simulink model "TEST_LIDAR"  (R2022b)
settings: Solver=FixedStepAuto  StartTime=0.0  StopTime=inf  FixedStep=1e-3  RelTol=1e-3  EnableMultiTasking=on
model workspace (MAT data in the model file):
  SL_ROS_VariableLengthArrays_MaxSizes : object (value not decoded)
values from neighbouring files (symbols this model uses):
  data = theClient.GetLastFrameOfData()    [FuncMotive.m]
undefined symbols (not defined in the file or in its folder): angular, carstamp, CIRCUIT, CLTF_DAMP, CLTF_FREQ, CLTF_GAIN, CONTROL, CONTROL_INI, DiscIntNeverNeededParam, INPUT, linear, MCP3201, MD25, MODEL, MODEL_INI, mpcstate, MPU60X0, MPU9250, MSG, NAV_MPC_CONTROL, OUTPUT, RCRX, SAMPLING_TIME, SYSID_INPUT, VL6180X
libraries: raspberrypiCommlib x160, simulink x89, raspberrypiNetworklib x22, ros2lib x14, dspsigattribs x14, embedlinuxBasiclib x12, ctrlSharedLib x2, mpclib x1, vrlib x1, sldrtlib x1
(part 4 of 19)

== system TEST_LIDAR/GAZEBO SIMULATION/COMMUNICATIONS/TCP//IP NAV ==
  Bus Selector : BusSelector  OutputSignals=INPUT.NAV_EARTH_POS,INPUT.NAV_EULER_ANG
  Data Store Read2 : DataStoreRead  DataStoreName=CONTROL  SampleTime=SAMPLING_TIME  IndexOptions=Index vector (dialog)  Indices=1  OutputSizes=1
  Data Store Write1 : DataStoreWrite  DataStoreName=CONTROL  DataStoreElements=CONTROL.STATE.NAV_RX_STATUS  IndexOptions=Index vector (dialog)  Indices=1  OutputSizes=1
  Data Store Write2 : DataStoreWrite  DataStoreName=CONTROL  IndexOptions=Index vector (dialog)  Indices=1  OutputSizes=1
  Data Type Conversion : DataTypeConversion  OutDataTypeStr=uint8  SaturateOnIntegerOverflow=off  RndMeth=Floor
  Display{,1..3} (4 alike) : Display
  NAV RX : MATLAB Function  Priority=20  TreatAsAtomicUnit=on
  NAV_EARTH_POS : Scope
  NAV_EULER_ANG : Scope
  TCP/IP Receive : raspberrypiNetworklib/TCP//IP Receive  Mode_=Server  LocalServerPort_=3000  RemoteAddr_=127.0.0.1  RemoteServerPort_=3000  DataType_=uint8  DataSize_=24  SampleTime_=SAMPLING_TIME  SimulateUsing=Code generation  ClientPortBindingSelection_=off  ClientPortToBind_=35000  BlockingMode_=off  BlockTimeout_=0.1  BlockPlatform=RASPBERRYPI
  wires:
  NAV RX/1(CONTROL) -> Bus Selector/1, Data Store Write2/1
  Data Store Read2/1 -> NAV RX/1(CONTROL_IN)
  TCP/IP Receive/1 -> NAV RX/2(PAYLOAD), Display1/1
  Bus Selector/1 -> NAV_EARTH_POS/1, Display2/1  "<NAV_EARTH_POS>"
  Bus Selector/2 -> NAV_EULER_ANG/1, Display3/1  "<NAV_EULER_ANG>"
  Data Type Conversion/1 -> Data Store Write1/1, Display/1, NAV RX/3(STATUS)
  TCP/IP Receive/2 -> Data Type Conversion/1

== system TEST_LIDAR/GAZEBO SIMULATION/COMMUNICATIONS/TCP//IP SLAM ==
  Data Store Read1 : DataStoreRead  DataStoreName=CONTROL  SampleTime=SAMPLING_TIME  IndexOptions=Index vector (dialog)  Indices=1  OutputSizes=1
  SLAM TX : MATLAB Function  Priority=20  TreatAsAtomicUnit=on
  TCP/IP Send : raspberrypiNetworklib/TCP//IP Send  Mode_=Server  LocalServerPort_=7001  RemoteAddr_=127.0.0.1  RemoteServerPort_=25000  SimulateUsing=Code generation  ClientPortBindingSelection_=off  ClientPortToBind_=35000  BlockingMode_=off  BlockTimeout_=0.1  BlockPlatform=RASPBERRYPI
  wires:
  SLAM TX/1(PAYLOAD) -> TCP/IP Send/1
  Data Store Read1/1 -> SLAM TX/1(CONTROL)

== system TEST_LIDAR/GAZEBO SIMULATION/COMMUNICATIONS/TCP//IP TEST ==
  Constant : Constant  Value=127  OutDataTypeStr=uint8  SampleTime=SAMPLING_TIME
  Data Type Conversion : DataTypeConversion  OutDataTypeStr=uint8  SaturateOnIntegerOverflow=off  RndMeth=Floor
  Display2 : Display
  Display3 : Display
  TCP/IP Receive : raspberrypiNetworklib/TCP//IP Receive  Mode_=Client  LocalServerPort_=3000  RemoteAddr_=192.168.1.21  RemoteServerPort_=27000  DataType_=uint8  DataSize_=1  SampleTime_=SAMPLING_TIME  SimulateUsing=Code generation  ClientPortBindingSelection_=off  ClientPortToBind_=35000  BlockingMode_=off  BlockTimeout_=0.1  BlockPlatform=RASPBERRYPI
  TCP/IP Send : raspberrypiNetworklib/TCP//IP Send  Mode_=Server  LocalServerPort_=27000  RemoteAddr_=127.0.0.1  RemoteServerPort_=25000  SimulateUsing=Code generation  ClientPortBindingSelection_=off  ClientPortToBind_=35000  BlockingMode_=off  BlockTimeout_=0.1  BlockPlatform=RASPBERRYPI
  wires:
  TCP/IP Receive/2 -> Data Type Conversion/1
  Data Type Conversion/1 -> Display3/1
  Constant/1 -> TCP/IP Send/1
  TCP/IP Receive/1 -> Display2/1

== system TEST_LIDAR/GAZEBO SIMULATION/COMMUNICATIONS/UART ==
  Compare To Zero : simulink/Logic and Bit Operations/Compare To Zero  relop=>  OutDataTypeStr=boolean
  Data Store Read : DataStoreRead  DataStoreName=CONTROL  SampleTime=SAMPLING_TIME  DataStoreElements=CONTROL.STATE.UART_MODE  IndexOptions=Index vector (dialog)  Indices=1  OutputSizes=1
  MSG_RX : Subsystem  Priority=10
      settings: RTWSystemCode=Nonreusable function  FunctionWithSeparateData=on
  MSG_TX : Subsystem  Priority=10
      settings: RTWSystemCode=Nonreusable function  FunctionWithSeparateData=on
  wires:
  Data Store Read/1 -> Compare To Zero/1
  Compare To Zero/1 -> MSG_TX/Enable

== system TEST_LIDAR/GAZEBO SIMULATION/COMMUNICATIONS/UART_MUX ==
  A : embedlinuxBasiclib/GPIO Write  Priority=4  board=Pi 3 Model B+  gpio=8  direction=Output  blockPlatform=Raspberry Pi
  B : embedlinuxBasiclib/GPIO Write  Priority=5  board=Pi 3 Model B+  gpio=18  direction=Output  blockPlatform=Raspberry Pi
  BT MCS : Subsystem  Priority=1
      settings: RTWSystemCode=Nonreusable function  FunctionWithSeparateData=on
  INH : embedlinuxBasiclib/GPIO Write  Priority=6  board=Pi 3 Model B+  gpio=5  direction=Output  blockPlatform=Raspberry Pi
  MATLAB Function : MATLAB Function  Priority=3  TreatAsAtomicUnit=on
  RCRX iBUS : Subsystem  Priority=2
  Serial Read : raspberrypiCommlib/Serial Read  Priority=0  board=Pi 3 Model B+  SCIModule_=/dev/ttyS0  Baudrate_=57600  Parity=None  StopBits_=1  HardwareFlowControl=None  ByteOrder=LittleEndian  DataLength=50  DataType=uint8  OutputStatus=on  SampleTime=SAMPLING_TIME  blockPlatform=RaspberryPi
  Terminator : Terminator
  wires:
  Serial Read/1 -> BT MCS/1(Data), RCRX iBUS/1(Data)
  Serial Read/2 -> Terminator/1
  MATLAB Function/5(BL) -> BT MCS/Enable
  MATLAB Function/4(RCRX) -> RCRX iBUS/Enable
  MATLAB Function/3(INH) -> INH/1
  MATLAB Function/2(B) -> B/1
  MATLAB Function/1(A) -> A/1

== system TEST_LIDAR/GAZEBO SIMULATION/COMMUNICATIONS/UDP//ROS ==
  Compare To Zero : simulink/Logic and Bit Operations/Compare To Zero  relop=>  OutDataTypeStr=boolean
  Data Store Read : DataStoreRead  DataStoreName=MSG  SampleTime=SAMPLING_TIME  DataStoreElements=MSG.TX_BUFFER(1,1)  IndexOptions=Index vector (dialog)  Indices=1  OutputSizes=1
  MSG_RX : Subsystem  Priority=10  TreatAsAtomicUnit=on
      settings: RTWSystemCode=Nonreusable function  FunctionWithSeparateData=on
  MSG_TX : Subsystem  Priority=10
      settings: RTWSystemCode=Nonreusable function  FunctionWithSeparateData=on
  wires:
  Compare To Zero/1 -> MSG_TX/Enable
  Data Store Read/1 -> Compare To Zero/1

== system TEST_LIDAR/GAZEBO SIMULATION/SENSORS/READ IMU ==
  " LPF 3" : Subsystem
  " LPF 4" : Subsystem
  Bus Selector : BusSelector  OutputSignals=linear_acceleration.x,linear_acceleration.y,linear_acceleration.z,angular_velocity.x,angular_velocity.y,angular_velocity.z
  Constant2 : Constant  Value=MPU60X0.ACCEL_CALIB  SampleTime=MPU60X0.SAMPLING_TIME
  Constant3 : Constant  Value=CONTROL_INI.PARAM.GRAVITY  SampleTime=MPU60X0.SAMPLING_TIME
  Constant4 : Constant  Value=MPU60X0.ALFA_CALIB  SampleTime=MPU60X0.SAMPLING_TIME
  Data Store Memory1 : DataStoreMemory  Priority=10  DataStoreName=MPU60X0_PITCH_OFFS  ReadBeforeWriteMsg=warning  WriteAfterWriteMsg=warning  WriteAfterReadMsg=warning  ShowAdditionalParam=off  OutDataTypeStr=double
  Data Store Memory5 : DataStoreMemory  Priority=10  DataStoreName=MPU60X0_ACCEL_OFFS  ReadBeforeWriteMsg=warning  WriteAfterWriteMsg=warning  WriteAfterReadMsg=warning  InitialValue=zeros(3,1)  ShowAdditionalParam=off  OutDataTypeStr=double
  Data Store Memory6 : DataStoreMemory  Priority=10  DataStoreName=MPU60X0_GYRO_OFFS  ReadBeforeWriteMsg=warning  WriteAfterWriteMsg=warning  WriteAfterReadMsg=warning  InitialValue=zeros(3,1)  ShowAdditionalParam=off  OutDataTypeStr=double
  Data Store Read : DataStoreRead  DataStoreName=CONTROL  SampleTime=MPU60X0.SAMPLING_TIME  DataStoreElements=CONTROL.STATE.VEHICLE_MODE  IndexOptions=Index vector (dialog)  Indices=1  OutputSizes=1
  Data Store Read1 : DataStoreRead  DataStoreName=MPU60X0_PITCH_OFFS  SampleTime=MPU60X0.SAMPLING_TIME  IndexOptions=Index vector (dialog)  Indices=1  OutputSizes=1
  Data Store Read6 : DataStoreRead  DataStoreName=MPU60X0_ACCEL_OFFS  SampleTime=MPU60X0.SAMPLING_TIME  IndexOptions=Index vector (dialog)  Indices=1  OutputSizes=1
  Data Store Read8 : DataStoreRead  DataStoreName=MPU60X0_GYRO_OFFS  SampleTime=MPU60X0.SAMPLING_TIME  IndexOptions=Index vector (dialog)  Indices=1  OutputSizes=1
  Data Store Read9 : DataStoreRead  DataStoreName=CONTROL  SampleTime=MPU60X0.SAMPLING_TIME  IndexOptions=Index vector (dialog)  Indices=1  OutputSizes=1
  Data Store Write3 : DataStoreWrite  DataStoreName=MPU60X0_ACCEL_OFFS  IndexOptions=Index vector (dialog)  Indices=1  OutputSizes=1
  Data Store Write4 : DataStoreWrite  DataStoreName=MPU60X0_GYRO_OFFS  IndexOptions=Index vector (dialog)  Indices=1  OutputSizes=1
  Data Store Write5 : DataStoreWrite  DataStoreName=CONTROL  IndexOptions=Index vector (dialog)  Indices=1  OutputSizes=1
  FILTER POLE : Subsystem
  GRAVITY ROTATION : MATLAB Function  TreatAsAtomicUnit=on
  IMU CALIBRATION : MATLAB Function  Priority=30  TreatAsAtomicUnit=on
  LPF 1 : Subsystem
  "LPF 2 " : Subsystem
  MEAN FILTER : DiscreteFilter  Numerator=1/floor(SAMPLING_TIME*1000)*ones(1,floor(SAMPLING_TIME*1000))  Denominator=[1 zeros(1,floor(SAMPLING_TIME*1000)-1)]
  "MEAN FILTER " : DiscreteFilter  Numerator=1/floor(SAMPLING_TIME*1000)*ones(1,floor(SAMPLING_TIME*1000))  Denominator=[1 zeros(1,floor(SAMPLING_TIME*1000)-1)]
  Mux : Mux  Inputs=3
  Mux1 : Mux  Inputs=3
  Scope : Scope  NumInputPorts=2
  Subscribe : ros2lib/Subscribe  topicSource=Specify your own  topic=/imu  messageType=sensor_msgs/Imu  sampleTime=-1  QOSHistory=Keep last  QOSDepth=1  QOSReliability=Reliable  QOSDurability=Volatile
      settings: LibrarySourceBlock=roslib/ROS 2/Subscribe
  Terminator : Terminator
  wires:
  Constant4/1 -> IMU CALIBRATION/11(ALFA_CALIB)
  Constant2/1 -> IMU CALIBRATION/10(ACCEL_CALIB)
  FILTER POLE/1(ALFA) -> " LPF 4"/2(ALFA), " LPF 3"/2(ALFA), LPF 1/2(ALFA), "LPF 2 "/2(ALFA)
  Mux1/1 -> "MEAN FILTER "/1, IMU CALIBRATION/6(GYRO), " LPF 3"/1(IN), Scope/2
  LPF 1/1(OUT) -> IMU CALIBRATION/3(ACCEL_FILT)
  " LPF 3"/1(OUT) -> IMU CALIBRATION/7(GYRO_FILT)
  " LPF 4"/1(OUT) -> IMU CALIBRATION/9(GYRO_MEAN_FILT)
  Data Store Read9/1 -> IMU CALIBRATION/1(CONTROL_IN)
  "LPF 2 "/1(OUT) -> IMU CALIBRATION/5(ACCEL_MEAN_FILT)
  IMU CALIBRATION/3(GYRO_OFFS_OUT) -> Data Store Write4/1
  Data Store Read6/1 -> IMU CALIBRATION/12(ACCEL_OFFS_IN)
  IMU CALIBRATION/1(CONTROL) -> Data Store Write5/1
  MEAN FILTER/1 -> "LPF 2 "/1(IN), IMU CALIBRATION/4(ACCEL_MEAN)
  Data Store Read8/1 -> IMU CALIBRATION/13(GYRO_OFFS_IN)
  IMU CALIBRATION/2(ACCEL_OFFS_OUT) -> Data Store Write3/1
  "MEAN FILTER "/1 -> IMU CALIBRATION/8(GYRO_MEAN), " LPF 4"/1(IN)
  Mux/1 -> Scope/1, IMU CALIBRATION/2(ACCEL), LPF 1/1(IN), MEAN FILTER/1
  Constant3/1 -> GRAVITY ROTATION/2(GRAVITY)
  Data Store Read1/1 -> GRAVITY ROTATION/1(PITCH_OFFSET)
  GRAVITY ROTATION/1(GRAVITY_VECTOR) -> IMU CALIBRATION/14(GRAVITY_VECTOR)
  Data Store Read/1 -> GRAVITY ROTATION/3(VEHICLE_MODE)
  Subscribe/2 -> Bus Selector/1
  Subscribe/1 -> Terminator/1
  Bus Selector/1 -> Mux/1  "<x>"
  Bus Selector/2 -> Mux/2  "<y>"
  Bus Selector/3 -> Mux/3  "<z>"
  Bus Selector/4 -> Mux1/1  "<x>"
  Bus Selector/5 -> Mux1/2  "<y>"
  Bus Selector/6 -> Mux1/3  "<z>"

== system TEST_LIDAR/GAZEBO SIMULATION/SENSORS/READ MOTOR ENCODER ==
  Bus Selector : BusSelector  OutputSignals=data
  Bus Selector1 : BusSelector  OutputSignals=data
  Bus Selector2 : BusSelector  OutputSignals=INPUT.FORWARD_VEL,INPUT.YAW_RATE
  Data Store Read : DataStoreRead  DataStoreName=CONTROL  SampleTime=SAMPLING_TIME  IndexOptions=Index vector (dialog)  Indices=1  OutputSizes=1
  Data Store Write1 : DataStoreWrite  DataStoreName=CONTROL  IndexOptions=Index vector (dialog)  Indices=1  OutputSizes=1
  MATLAB Function : MATLAB Function  TreatAsAtomicUnit=on
  Mux : Mux  Inputs=2
  Mux1 : Mux  Inputs=2
  READ_ENCODER : MATLAB Function  TreatAsAtomicUnit=on
  Scope : Scope  NumInputPorts=3
  Subscribe : ros2lib/Subscribe  topicSource=Select from ROS network  topic=/model/FullKitt/right_wheel_joint/motor_encoder  messageType=std_msgs/Int32  sampleTime=-1  QOSHistory=Keep last  QOSDepth=1  QOSReliability=Reliable  QOSDurability=Volatile
      settings: LibrarySourceBlock=roslib/ROS 2/Subscribe
  Subscribe1 : ros2lib/Subscribe  topicSource=Select from ROS network  topic=/model/FullKitt/left_wheel_joint/motor_encoder  messageType=std_msgs/Int32  sampleTime=-1  QOSHistory=Keep last  QOSDepth=1  QOSReliability=Reliable  QOSDurability=Volatile
      settings: LibrarySourceBlock=roslib/ROS 2/Subscribe
  wires:
  Data Store Read/1 -> READ_ENCODER/1(CONTROL_IN)
  READ_ENCODER/1(CONTROL) -> Bus Selector2/1, Data Store Write1/1
  Subscribe/2 -> Bus Selector/1
  Subscribe1/2 -> Bus Selector1/1
  Bus Selector/1 -> MATLAB Function/1(right_enc), Mux/1, READ_ENCODER/2(right_enc)  "<data>"
  Bus Selector1/1 -> MATLAB Function/2(left_enc), Mux/2, READ_ENCODER/3(left_enc)  "<data>"
  Bus Selector2/1 -> Mux1/2  "<FORWARD_VEL>"
  Bus Selector2/2 -> Scope/2  "<YAW_RATE>"
  Mux/1 -> Scope/3
  Mux1/1 -> Scope/1
  MATLAB Function/1(avg_encoder) -> Mux1/1

== system TEST_LIDAR/GAZEBO SIMULATION/SENSORS/WALL RANGE SENSOR ==
  ANGLE AND DISTANCE COMPUTATION : Subsystem  TreatAsAtomicUnit=on
      settings: MinAlgLoopOccurrences=on
  Data Store Memory : DataStoreMemory  DataStoreName=REAR_DISTANCE  ReadBeforeWriteMsg=warning  WriteAfterWriteMsg=warning  WriteAfterReadMsg=warning  ShowAdditionalParam=off  OutDataTypeStr=double
  Data Store Memory1 : DataStoreMemory  DataStoreName=FRONT_DISTANCE  ReadBeforeWriteMsg=warning  WriteAfterWriteMsg=warning  WriteAfterReadMsg=warning  ShowAdditionalParam=off  OutDataTypeStr=double
  FRONT : Subsystem  TreatAsAtomicUnit=on
      settings: MinAlgLoopOccurrences=on  RTWSystemCode=Nonreusable function  FunctionWithSeparateData=on
  REAR : Subsystem  TreatAsAtomicUnit=on
      settings: MinAlgLoopOccurrences=on  RTWSystemCode=Nonreusable function  FunctionWithSeparateData=on

== system TEST_LIDAR/HARDWARE/ACTUATORS/MD25_I2C ==
  Cast : DataTypeConversion  OutDataTypeStr=uint8  SaturateOnIntegerOverflow=off  RndMeth=Floor
  Compare To Constant : simulink/Logic and Bit Operations/Compare To Constant  relop===  const=0  OutDataTypeStr=uint8
  Data Store Memory : DataStoreMemory  Priority=10  DataStoreName=MD25_INIT  ReadBeforeWriteMsg=warning  WriteAfterWriteMsg=warning  WriteAfterReadMsg=warning  ShowAdditionalParam=off  OutDataTypeStr=boolean
  Data Store Read : DataStoreRead  DataStoreName=MD25_INIT  SampleTime=SAMPLING_TIME  IndexOptions=Index vector (dialog)  Indices=1  OutputSizes=1
  Data Store Read1 : DataStoreRead  DataStoreName=MD25_INIT  IndexOptions=Index vector (dialog)  Indices=1  OutputSizes=1
  Data Store Read2 : DataStoreRead  DataStoreName=CONTROL  SampleTime=SAMPLING_TIME  DataStoreElements=CONTROL.STATE.CURRENT_STATUS_SYS  IndexOptions=Index vector (dialog)  Indices=1  OutputSizes=1
  Data Store Write : DataStoreWrite  DataStoreName=CONTROL  DataStoreElements=CONTROL.STATE.MD25_INIT  IndexOptions=Index vector (dialog)  Indices=1  OutputSizes=1
  Logical Operator : Logic  Operator=NOT  AllPortsSameDT=off  OutDataTypeStr=boolean
  MD25 INITIALIZATION : Subsystem  Priority=10
      settings: RTWSystemCode=Nonreusable function
  READ BATTERY VOLTAGE : Subsystem  Priority=20  TreatAsAtomicUnit=on
      settings: RTWSystemCode=Nonreusable function
  READ MOTOR CURRENT : Subsystem  Priority=30  TreatAsAtomicUnit=on
      settings: RTWSystemCode=Nonreusable function
  READ MOTOR ENCODER : Subsystem  Priority=40  TreatAsAtomicUnit=on
      settings: RTWSystemCode=Nonreusable function
  RESET MOTOR ENCODER : Subsystem  Priority=50  TreatAsAtomicUnit=on
      settings: RTWSystemCode=Nonreusable function
  "WRITE PWM MOTOR " : Subsystem  Priority=50  TreatAsAtomicUnit=on
      settings: RTWSystemCode=Nonreusable function
  wires:
  Logical Operator/1 -> MD25 INITIALIZATION/Enable
  Data Store Read1/1 -> Cast/1
  Cast/1 -> Data Store Write/1
  Data Store Read/1 -> "WRITE PWM MOTOR "/Enable, READ MOTOR ENCODER/Enable, READ MOTOR CURRENT/Enable, READ BATTERY VOLTAGE/Enable, Logical Operator/1
  Data Store Read2/1 -> Compare To Constant/1
  Compare To Constant/1 -> RESET MOTOR ENCODER/Enable

== system TEST_LIDAR/HARDWARE/ACTUATORS/RGB ==
  BLUE : embedlinuxBasiclib/GPIO Write  board=Pi 3 Model B+  gpio=25  direction=Output  blockPlatform=Raspberry Pi
  Cast1 : DataTypeConversion  OutDataTypeStr=boolean  SaturateOnIntegerOverflow=off  RndMeth=Floor
  Cast2 : DataTypeConversion  OutDataTypeStr=boolean  SaturateOnIntegerOverflow=off  RndMeth=Floor
  Cast3 : DataTypeConversion  OutDataTypeStr=boolean  SaturateOnIntegerOverflow=off  RndMeth=Floor
  Data Store Read : DataStoreRead  DataStoreName=CONTROL  SampleTime=SAMPLING_TIME  DataStoreElements=CONTROL.OUTPUT.LEDS(:,:)  IndexOptions=Index vector (dialog)  Indices=1  OutputSizes=1
  Demux : Demux  Outputs=3
  GREEN : embedlinuxBasiclib/GPIO Write  board=Pi 3 Model B+  gpio=24  direction=Output  blockPlatform=Raspberry Pi
  RED : embedlinuxBasiclib/GPIO Write  board=Pi 3 Model B+  gpio=23  direction=Output  blockPlatform=Raspberry Pi
  wires:
  Data Store Read/1 -> Demux/1
  Demux/1 -> Cast1/1
  Demux/2 -> Cast2/1
  Demux/3 -> Cast3/1
  Cast1/1 -> RED/1
  Cast2/1 -> GREEN/1
  Cast3/1 -> BLUE/1

== system TEST_LIDAR/HARDWARE/COMMUNICATIONS/BT_RX ==
  Bus Selector : BusSelector  OutputSignals=INPUT.MCS_EARTH_POS,INPUT.MCS_EULER_ANG
  Data Store Read2 : DataStoreRead  DataStoreName=CONTROL  SampleTime=SAMPLING_TIME  IndexOptions=Index vector (dialog)  Indices=1  OutputSizes=1
  Data Store Write1 : DataStoreWrite  DataStoreName=CONTROL  DataStoreElements=CONTROL.STATE.MCS_RX_STATUS  IndexOptions=Index vector (dialog)  Indices=1  OutputSizes=1
  Data Store Write2 : DataStoreWrite  DataStoreName=CONTROL  IndexOptions=Index vector (dialog)  Indices=1  OutputSizes=1
  Data Type Conversion : DataTypeConversion  OutDataTypeStr=uint8  SaturateOnIntegerOverflow=off  RndMeth=Floor
  Display{,1..3} (4 alike) : Display
  MCS RX : MATLAB Function  Priority=20  TreatAsAtomicUnit=on
  MCS_EARTH_POS : Scope
  MCS_EULER_ANG : Scope
  Serial Read : raspberrypiCommlib/Serial Read  board=Pi 3 Model B+  SCIModule_=/dev/ttyUSB0  Baudrate_=115200  Parity=None  StopBits_=1  HardwareFlowControl=None  ByteOrder=LittleEndian  DataLength=50  DataType=uint8  OutputStatus=on  SampleTime=SAMPLING_TIME  blockPlatform=RaspberryPi
  wires:
  MCS RX/1(CONTROL) -> Bus Selector/1, Data Store Write2/1
  Data Store Read2/1 -> MCS RX/1(CONTROL_IN)
  Serial Read/1 -> Display1/1, MCS RX/2(BUFFER_RX_LAST)
  Serial Read/2 -> Data Type Conversion/1
  Bus Selector/1 -> MCS_EARTH_POS/1, Display2/1  "<MCS_EARTH_POS>"
  Bus Selector/2 -> MCS_EULER_ANG/1, Display3/1  "<MCS_EULER_ANG>"
  Data Type Conversion/1 -> Data Store Write1/1, Display/1, MCS RX/3(STATUS)

== system TEST_LIDAR/HARDWARE/COMMUNICATIONS/TCP//IP ==
  Compare To Zero : simulink/Logic and Bit Operations/Compare To Zero  relop=>  OutDataTypeStr=boolean
  Data Store Read : DataStoreRead  DataStoreName=MSG  SampleTime=SAMPLING_TIME  DataStoreElements=MSG.TX_BUFFER(1,1)  IndexOptions=Index vector (dialog)  Indices=1  OutputSizes=1
  MSG_RX : Subsystem  Priority=10  TreatAsAtomicUnit=on
      settings: RTWSystemCode=Nonreusable function  FunctionWithSeparateData=on
  MSG_TX : Subsystem  Priority=10
      settings: RTWSystemCode=Nonreusable function  FunctionWithSeparateData=on
  wires:
  Compare To Zero/1 -> MSG_TX/Enable
  Data Store Read/1 -> Compare To Zero/1

== system TEST_LIDAR/HARDWARE/COMMUNICATIONS/TCP//IP LIDAR ==
  Bus Selector : BusSelector  OutputSignals=INPUT.LIDAR_2D
  Data Store Read1 : DataStoreRead  DataStoreName=CONTROL  SampleTime=SAMPLING_TIME  DataStoreElements=CONTROL.STATE.LIDAR_2D_MODE  IndexOptions=Index vector (dialog)  Indices=1  OutputSizes=1
  Data Store Read2 : DataStoreRead  DataStoreName=CONTROL  SampleTime=SAMPLING_TIME  IndexOptions=Index vector (dialog)  Indices=1  OutputSizes=1
  Data Store Write1 : DataStoreWrite  DataStoreName=CONTROL  DataStoreElements=CONTROL.STATE.NAV_RX_STATUS  IndexOptions=Index vector (dialog)  Indices=1  OutputSizes=1
  Data Store Write2 : DataStoreWrite  DataStoreName=CONTROL  IndexOptions=Index vector (dialog)  Indices=1  OutputSizes=1
  Data Type Conversion : DataTypeConversion  OutDataTypeStr=uint8  SaturateOnIntegerOverflow=off  RndMeth=Floor
  Display : Display
  Display1 : Display
  Display2 : Display
  NAV RX : MATLAB Function  Priority=20  TreatAsAtomicUnit=on
  TCP/IP Receive : raspberrypiNetworklib/TCP//IP Receive  Mode_=Server  LocalServerPort_=7000  RemoteAddr_=127.0.0.1  RemoteServerPort_=3000  DataType_=uint8  DataSize_=160  SampleTime_=SAMPLING_TIME  SimulateUsing=Code generation  ClientPortBindingSelection_=off  ClientPortToBind_=35000  BlockingMode_=off  BlockTimeout_=0.1  BlockPlatform=RASPBERRYPI
  TCP/IP Send : raspberrypiNetworklib/TCP//IP Send  Mode_=Server  LocalServerPort_=7001  RemoteAddr_=127.0.0.1  RemoteServerPort_=25000  SimulateUsing=Code generation  ClientPortBindingSelection_=off  ClientPortToBind_=35000  BlockingMode_=off  BlockTimeout_=0.1  BlockPlatform=RASPBERRYPI
  wires:
  NAV RX/1(CONTROL) -> Bus Selector/1, Data Store Write2/1
  Data Store Read2/1 -> NAV RX/1(CONTROL_IN)
  TCP/IP Receive/1 -> NAV RX/2(PAYLOAD), Display1/1
  Bus Selector/1 -> Display2/1  "<LIDAR_2D>"
  Data Type Conversion/1 -> Data Store Write1/1, Display/1, NAV RX/3(STATUS)
  TCP/IP Receive/2 -> Data Type Conversion/1
  Data Store Read1/1 -> TCP/IP Send/1

== system TEST_LIDAR/HARDWARE/COMMUNICATIONS/TCP//IP MCS ==
  Bus Selector : BusSelector  OutputSignals=INPUT.MCS_EARTH_POS,INPUT.MCS_EULER_ANG
  Data Store Read2 : DataStoreRead  DataStoreName=CONTROL  SampleTime=SAMPLING_TIME  IndexOptions=Index vector (dialog)  Indices=1  OutputSizes=1
  Data Store Write1 : DataStoreWrite  DataStoreName=CONTROL  DataStoreElements=CONTROL.STATE.MCS_RX_STATUS  IndexOptions=Index vector (dialog)  Indices=1  OutputSizes=1
  Data Store Write2 : DataStoreWrite  DataStoreName=CONTROL  IndexOptions=Index vector (dialog)  Indices=1  OutputSizes=1
  Data Type Conversion : DataTypeConversion  OutDataTypeStr=uint8  SaturateOnIntegerOverflow=off  RndMeth=Floor
  Display{,1..3} (4 alike) : Display
  MCS RX : MATLAB Function  Priority=20  TreatAsAtomicUnit=on
  MCS_EARTH_POS : Scope
  MCS_EULER_ANG : Scope
  TCP/IP Receive : raspberrypiNetworklib/TCP//IP Receive  Mode_=Server  LocalServerPort_=15000  RemoteAddr_=127.0.0.1  RemoteServerPort_=3000  DataType_=uint8  DataSize_=26  SampleTime_=SAMPLING_TIME  SimulateUsing=Code generation  ClientPortBindingSelection_=off  ClientPortToBind_=35000  BlockingMode_=off  BlockTimeout_=0.1  BlockPlatform=RASPBERRYPI
  wires:
  TCP/IP Receive/2 -> Data Type Conversion/1
  Data Type Conversion/1 -> MCS RX/3(STATUS), Display/1, Data Store Write1/1
  Bus Selector/2 -> Display3/1, MCS_EULER_ANG/1  "<MCS_EULER_ANG>"
  Bus Selector/1 -> Display2/1, MCS_EARTH_POS/1  "<MCS_EARTH_POS>"
  TCP/IP Receive/1 -> Display1/1, MCS RX/2(PAYLOAD)
  Data Store Read2/1 -> MCS RX/1(CONTROL_IN)
  MCS RX/1(CONTROL) -> Data Store Write2/1, Bus Selector/1

== system TEST_LIDAR/HARDWARE/COMMUNICATIONS/TCP//IP NAV ==
  Bus Selector : BusSelector  OutputSignals=INPUT.NAV_EARTH_POS,INPUT.NAV_EULER_ANG
  Data Store Read2 : DataStoreRead  DataStoreName=CONTROL  SampleTime=SAMPLING_TIME  IndexOptions=Index vector (dialog)  Indices=1  OutputSizes=1
  Data Store Write1 : DataStoreWrite  DataStoreName=CONTROL  DataStoreElements=CONTROL.STATE.NAV_RX_STATUS  IndexOptions=Index vector (dialog)  Indices=1  OutputSizes=1
  Data Store Write2 : DataStoreWrite  DataStoreName=CONTROL  IndexOptions=Index vector (dialog)  Indices=1  OutputSizes=1
  Data Type Conversion : DataTypeConversion  OutDataTypeStr=uint8  SaturateOnIntegerOverflow=off  RndMeth=Floor
  Display{,1..3} (4 alike) : Display
  NAV RX : MATLAB Function  Priority=20  TreatAsAtomicUnit=on
  NAV_EARTH_POS : Scope
  NAV_EULER_ANG : Scope
  TCP/IP Receive : raspberrypiNetworklib/TCP//IP Receive  Mode_=Server  LocalServerPort_=3000  RemoteAddr_=127.0.0.1  RemoteServerPort_=3000  DataType_=uint8  DataSize_=24  SampleTime_=SAMPLING_TIME  SimulateUsing=Code generation  ClientPortBindingSelection_=off  ClientPortToBind_=35000  BlockingMode_=off  BlockTimeout_=0.1  BlockPlatform=RASPBERRYPI
  wires:
  NAV RX/1(CONTROL) -> Bus Selector/1, Data Store Write2/1
  Data Store Read2/1 -> NAV RX/1(CONTROL_IN)
  TCP/IP Receive/1 -> NAV RX/2(PAYLOAD), Display1/1
  Bus Selector/1 -> NAV_EARTH_POS/1, Display2/1  "<NAV_EARTH_POS>"
  Bus Selector/2 -> NAV_EULER_ANG/1, Display3/1  "<NAV_EULER_ANG>"
  Data Type Conversion/1 -> Data Store Write1/1, Display/1, NAV RX/3(STATUS)
  TCP/IP Receive/2 -> Data Type Conversion/1

== system TEST_LIDAR/HARDWARE/COMMUNICATIONS/TCP//IP RPI4 ==
  Bus Selector : BusSelector  OutputSignals=INPUT.LIDAR_2D
  Bus Selector1 : BusSelector  OutputSignals=PARAM.LIDAR_2D_MAP
  Data Store Read2 : DataStoreRead  Priority=10  DataStoreName=CONTROL  SampleTime=SAMPLING_TIME  IndexOptions=Index vector (dialog)  Indices=1  OutputSizes=1
  Data Store Read3 : DataStoreRead  Priority=40  DataStoreName=CONTROL  SampleTime=SAMPLING_TIME  IndexOptions=Index vector (dialog)  Indices=1  OutputSizes=1
  Data Store Write1 : DataStoreWrite  DataStoreName=CONTROL  DataStoreElements=CONTROL.STATE.NAV_RX_STATUS  IndexOptions=Index vector (dialog)  Indices=1  OutputSizes=1
  Data Store Write2 : DataStoreWrite  Priority=30  DataStoreName=CONTROL  IndexOptions=Index vector (dialog)  Indices=1  OutputSizes=1
  Data Type Conversion : DataTypeConversion  OutDataTypeStr=uint8  SaturateOnIntegerOverflow=off  RndMeth=Floor
  Display : Display
  Display1 : Display
  Display2 : Display
  RPI4 CODER : MATLAB Function  Priority=50  TreatAsAtomicUnit=on
  RPI4 DECODER : MATLAB Function  Priority=20  TreatAsAtomicUnit=on
  Scope : Scope
  TCP/IP Receive : raspberrypiNetworklib/TCP//IP Receive  Priority=0  Mode_=Server  LocalServerPort_=7000  RemoteAddr_=127.0.0.1  RemoteServerPort_=3000  DataType_=uint8  DataSize_=584  SampleTime_=SAMPLING_TIME  SimulateUsing=Code generation  ClientPortBindingSelection_=off  ClientPortToBind_=35000  BlockingMode_=off  BlockTimeout_=0.1  BlockPlatform=RASPBERRYPI
  TCP/IP Send : raspberrypiNetworklib/TCP//IP Send  Priority=60  Mode_=Server  LocalServerPort_=7001  RemoteAddr_=127.0.0.1  RemoteServerPort_=25000  SimulateUsing=Code generation  ClientPortBindingSelection_=off  ClientPortToBind_=35000  BlockingMode_=off  BlockTimeout_=0.1  BlockPlatform=RASPBERRYPI
  wires:
  TCP/IP Receive/2 -> Data Type Conversion/1
  Data Type Conversion/1 -> RPI4 DECODER/3(STATUS), Display/1, Data Store Write1/1
  Bus Selector/1 -> Display2/1  "<LIDAR_2D>"
  TCP/IP Receive/1 -> RPI4 DECODER/2(RX_MSG), Display1/1
  Data Store Read2/1 -> RPI4 DECODER/1(CONTROL_IN)
  RPI4 CODER/1(TX_MSG) -> TCP/IP Send/1
  Data Store Read3/1 -> RPI4 CODER/1(CONTROL)
  RPI4 DECODER/1(CONTROL) -> Bus Selector1/1, Bus Selector/1, Data Store Write2/1
  Bus Selector1/1 -> Scope/1  "<LIDAR_2D_MAP>"

== system TEST_LIDAR/HARDWARE/COMMUNICATIONS/TCP//IP SLAM ==
  Data Store Read1 : DataStoreRead  DataStoreName=CONTROL  SampleTime=SAMPLING_TIME  IndexOptions=Index vector (dialog)  Indices=1  OutputSizes=1
  SLAM TX : MATLAB Function  Priority=20  TreatAsAtomicUnit=on
  TCP/IP Send : raspberrypiNetworklib/TCP//IP Send  Mode_=Server  LocalServerPort_=7001  RemoteAddr_=127.0.0.1  RemoteServerPort_=25000  SimulateUsing=Code generation  ClientPortBindingSelection_=off  ClientPortToBind_=35000  BlockingMode_=off  BlockTimeout_=0.1  BlockPlatform=RASPBERRYPI
  wires:
  SLAM TX/1(PAYLOAD) -> TCP/IP Send/1
  Data Store Read1/1 -> SLAM TX/1(CONTROL)

== system TEST_LIDAR/HARDWARE/COMMUNICATIONS/TCP//IP TEST ==
  Constant : Constant  Value=127  OutDataTypeStr=uint8  SampleTime=SAMPLING_TIME
  Data Type Conversion : DataTypeConversion  OutDataTypeStr=uint8  SaturateOnIntegerOverflow=off  RndMeth=Floor
  Display2 : Display
  Display3 : Display
  TCP/IP Receive : raspberrypiNetworklib/TCP//IP Receive  Mode_=Client  LocalServerPort_=3000  RemoteAddr_=192.168.1.21  RemoteServerPort_=27000  DataType_=uint8  DataSize_=1  SampleTime_=SAMPLING_TIME  SimulateUsing=Code generation  ClientPortBindingSelection_=off  ClientPortToBind_=35000  BlockingMode_=off  BlockTimeout_=0.1  BlockPlatform=RASPBERRYPI
  TCP/IP Send : raspberrypiNetworklib/TCP//IP Send  Mode_=Server  LocalServerPort_=27000  RemoteAddr_=127.0.0.1  RemoteServerPort_=25000  SimulateUsing=Code generation  ClientPortBindingSelection_=off  ClientPortToBind_=35000  BlockingMode_=off  BlockTimeout_=0.1  BlockPlatform=RASPBERRYPI
  wires:
  TCP/IP Receive/2 -> Data Type Conversion/1
  Data Type Conversion/1 -> Display3/1
  Constant/1 -> TCP/IP Send/1
  TCP/IP Receive/1 -> Display2/1

== system TEST_LIDAR/HARDWARE/COMMUNICATIONS/UART ==
  Compare To Zero : simulink/Logic and Bit Operations/Compare To Zero  relop=>  OutDataTypeStr=boolean
  Data Store Read : DataStoreRead  DataStoreName=CONTROL  SampleTime=SAMPLING_TIME  DataStoreElements=CONTROL.STATE.UART_MODE  IndexOptions=Index vector (dialog)  Indices=1  OutputSizes=1
  MSG_RX : Subsystem  Priority=10
      settings: RTWSystemCode=Nonreusable function  FunctionWithSeparateData=on
  MSG_TX : Subsystem  Priority=10
      settings: RTWSystemCode=Nonreusable function  FunctionWithSeparateData=on
  wires:
  Data Store Read/1 -> Compare To Zero/1
  Compare To Zero/1 -> MSG_TX/Enable

== system TEST_LIDAR/HARDWARE/COMMUNICATIONS/UART_MUX ==
  A : embedlinuxBasiclib/GPIO Write  Priority=4  board=Pi 3 Model B+  gpio=8  direction=Output  blockPlatform=Raspberry Pi
  B : embedlinuxBasiclib/GPIO Write  Priority=5  board=Pi 3 Model B+  gpio=18  direction=Output  blockPlatform=Raspberry Pi
  BT MCS : Subsystem  Priority=1
      settings: RTWSystemCode=Nonreusable function  FunctionWithSeparateData=on
  INH : embedlinuxBasiclib/GPIO Write  Priority=6  board=Pi 3 Model B+  gpio=5  direction=Output  blockPlatform=Raspberry Pi
  MATLAB Function : MATLAB Function  Priority=3  TreatAsAtomicUnit=on
  RCRX iBUS : Subsystem  Priority=2
  Serial Read : raspberrypiCommlib/Serial Read  Priority=0  board=Pi 3 Model B+  SCIModule_=/dev/ttyS0  Baudrate_=57600  Parity=None  StopBits_=1  HardwareFlowControl=None  ByteOrder=LittleEndian  DataLength=50  DataType=uint8  OutputStatus=on  SampleTime=SAMPLING_TIME  blockPlatform=RaspberryPi
  Terminator : Terminator
  wires:
  Serial Read/1 -> BT MCS/1(Data), RCRX iBUS/1(Data)
  Serial Read/2 -> Terminator/1
  MATLAB Function/5(BL) -> BT MCS/Enable
  MATLAB Function/4(RCRX) -> RCRX iBUS/Enable
  MATLAB Function/3(INH) -> INH/1
  MATLAB Function/2(B) -> B/1
  MATLAB Function/1(A) -> A/1

== system TEST_LIDAR/HARDWARE/COMMUNICATIONS/UDP//ROS ==
  Compare To Zero : simulink/Logic and Bit Operations/Compare To Zero  relop=>  OutDataTypeStr=boolean
  Data Store Read : DataStoreRead  DataStoreName=MSG  SampleTime=SAMPLING_TIME  DataStoreElements=MSG.TX_BUFFER(1,1)  IndexOptions=Index vector (dialog)  Indices=1  OutputSizes=1
  MSG_RX : Subsystem  Priority=10  TreatAsAtomicUnit=on
      settings: RTWSystemCode=Nonreusable function  FunctionWithSeparateData=on
  MSG_TX : Subsystem  Priority=10
      settings: RTWSystemCode=Nonreusable function  FunctionWithSeparateData=on
  wires:
  Compare To Zero/1 -> MSG_TX/Enable
  Data Store Read/1 -> Compare To Zero/1

== system TEST_LIDAR/HARDWARE/SENSORS/BUTTONS ==
  BUTTON A : embedlinuxBasiclib/GPIO Read  board=Pi 3 Model B+  gpio=4  internalResistor=Off  sampleTime=SAMPLING_TIME  direction=Input  blockPlatform=Raspberry Pi
  BUTTON B : embedlinuxBasiclib/GPIO Read  board=Pi 3 Model B+  gpio=13  internalResistor=Off  sampleTime=SAMPLING_TIME  direction=Input  blockPlatform=Raspberry Pi
  BUTTON C : embedlinuxBasiclib/GPIO Read  board=Pi 3 Model B+  gpio=22  internalResistor=Off  sampleTime=SAMPLING_TIME  direction=Input  blockPlatform=Raspberry Pi
  Cast : DataTypeConversion  OutDataTypeStr=uint8  SaturateOnIntegerOverflow=off  RndMeth=Floor
  Data Store Read1 : DataStoreRead  DataStoreName=CONTROL  SampleTime=SAMPLING_TIME  DataStoreElements=CONTROL.STATE.NAV_BUTTONS(:,:)  IndexOptions=Index vector (dialog)  Indices=1  OutputSizes=1
  Data Store Read5 : DataStoreRead  DataStoreName=CONTROL  SampleTime=SAMPLING_TIME  DataStoreElements=CONTROL.STATE.PC_BUTTONS(:,:)  IndexOptions=Index vector (dialog)  Indices=1  OutputSizes=1
  Data Store Write : DataStoreWrite  DataStoreName=CONTROL  DataStoreElements=CONTROL.STATE.BUTTONS(:,:)  IndexOptions=Index vector (dialog)  Indices=1  OutputSizes=1
  Data Type Conversion : DataTypeConversion  OutDataTypeStr=uint8  SaturateOnIntegerOverflow=off  RndMeth=Floor
  Display : Display
  Logical Operator : Logic  Operator=OR  Inputs=3  AllPortsSameDT=off
  Mux : Mux  Inputs=3
  wires:
  BUTTON A/1 -> Mux/1
  BUTTON B/1 -> Mux/2
  BUTTON C/1 -> Mux/3
  Mux/1 -> Display/1, Data Type Conversion/1
  Data Type Conversion/1 -> Logical Operator/1
  Logical Operator/1 -> Cast/1
  Data Store Read5/1 -> Logical Operator/2
  Cast/1 -> Data Store Write/1
  Data Store Read1/1 -> Logical Operator/3

== system TEST_LIDAR/HARDWARE/SENSORS/CURRENT_ADC_MCP3201_SPI ==
  ADC UPDATE : MATLAB Function  Priority=10  TreatAsAtomicUnit=on
  Bus Selector : BusSelector  OutputSignals=INPUT.CHARGING_CURRENT
  Constant : Constant  Value=[0 0 0 0]'  OutDataTypeStr=uint8  SampleTime=SAMPLING_TIME
  Constant1 : Constant  Value=MCP3201.NBITS  OutDataTypeStr=double  SampleTime=SAMPLING_TIME
  Constant2 : Constant  Value=MCP3201.R_SHUNT  OutDataTypeStr=double  SampleTime=SAMPLING_TIME
  Constant4 : Constant  Value=MCP3201.VREF  OutDataTypeStr=double  SampleTime=SAMPLING_TIME
  Data Store Read : DataStoreRead  DataStoreName=CONTROL  SampleTime=SAMPLING_TIME  IndexOptions=Index vector (dialog)  Indices=1  OutputSizes=1
  Data Store Write : DataStoreWrite  DataStoreName=CONTROL  IndexOptions=Index vector (dialog)  Indices=1  OutputSizes=1
  Data Type Conversion : DataTypeConversion  OutDataTypeStr=uint16  SaturateOnIntegerOverflow=off  RndMeth=Floor
  Demux : Demux
  Display : Display
  Display4 : Display
  Gain : Gain  Gain=256
  SPI Master Transfer : raspberrypiCommlib/SPI Master Transfer  BoardProperty=Pi 3 Model B  SSPin=SPI0_CE0  SPIModule=uint32(0)  Mode=Master  BusSpeed=1000000  Pin=SPI0_CE0  FirstBitToTransfer=Most significant bit (MSB)  ClockMode=0  BlockFunction=Transfer  RegisterAddress=0  OutputDataType=int8  OutputDataLength=1
  Scope : Scope
  Sum : Sum  Inputs=|++
  Terminator : Terminator
  Terminator1 : Terminator
  wires:
  Constant4/1 -> ADC UPDATE/2(VREF)
  Constant1/1 -> ADC UPDATE/3(NBITS)
  Bus Selector/1 -> Display4/1, Scope/1  "<CHARGING_CURRENT>"
  ADC UPDATE/1(CONTROL) -> Bus Selector/1, Data Store Write/1
  Data Store Read/1 -> ADC UPDATE/1(CONTROL_IN)
  Constant/1 -> SPI Master Transfer/1
  SPI Master Transfer/1 -> Demux/1, Display/1
  Demux/1 -> Terminator/1
  Demux/4 -> Terminator1/1
  Demux/2 -> Gain/1
  Gain/1 -> Sum/1
  Demux/3 -> Sum/2
  Sum/1 -> Data Type Conversion/1
  Data Type Conversion/1 -> ADC UPDATE/5(ADC_CODE)
  Constant2/1 -> ADC UPDATE/4(R_SHUNT)

== system TEST_LIDAR/HARDWARE/SENSORS/IMU MPU60X0_SPI ==
  Constant : Constant  Value=MPU60X0.FIFO_ENABLED  SampleTime=MPU60X0.SAMPLING_TIME
  Constant1 : Constant  Value=MPU60X0.TEMP_DIS  SampleTime=MPU60X0.SAMPLING_TIME
  Data Store Memory : DataStoreMemory  Priority=10  DataStoreName=MPU60X0_INIT  ReadBeforeWriteMsg=warning  WriteAfterWriteMsg=warning  WriteAfterReadMsg=warning  ShowAdditionalParam=off  OutDataTypeStr=boolean
  Data Store Read : DataStoreRead  DataStoreName=MPU60X0_INIT  SampleTime=MPU60X0.SAMPLING_TIME  IndexOptions=Index vector (dialog)  Indices=1  OutputSizes=1
  INITIALIZATION : Subsystem  Priority=0
      settings: RTWSystemCode=Nonreusable function
  Logical Operator : Logic  Operator=NOT  AllPortsSameDT=off  OutDataTypeStr=boolean
  Logical Operator1 : Logic  AllPortsSameDT=off  OutDataTypeStr=boolean
  Logical Operator2 : Logic  AllPortsSameDT=off  OutDataTypeStr=boolean
  Logical Operator3 : Logic  Operator=NOT  AllPortsSameDT=off  OutDataTypeStr=boolean
  Logical Operator4 : Logic  AllPortsSameDT=off  OutDataTypeStr=boolean
  Logical Operator5 : Logic  Operator=NOT  AllPortsSameDT=off  OutDataTypeStr=boolean
  READ FIFO : Subsystem  Priority=10  Commented=on  TreatAsAtomicUnit=on
      settings: RTWSystemCode=Nonreusable function
  READ IMU : Subsystem  Priority=20  TreatAsAtomicUnit=on
      settings: MinAlgLoopOccurrences=on  RTWSystemCode=Nonreusable function
  READ TEMP : Subsystem  Priority=30  Commented=on  TreatAsAtomicUnit=on
      settings: RTWSystemCode=Nonreusable function
  WHO_AM_I : Subsystem  Commented=on
  wires:
  Logical Operator/1 -> INITIALIZATION/Enable
  Data Store Read/1 -> WHO_AM_I/Enable, Logical Operator2/1, Logical Operator4/1, Logical Operator1/1, Logical Operator/1
  Logical Operator5/1 -> Logical Operator4/2
  Logical Operator3/1 -> Logical Operator2/2
  Constant1/1 -> Logical Operator3/1
  Logical Operator2/1 -> READ TEMP/Enable
  Constant/1 -> Logical Operator1/2, Logical Operator5/1
  Logical Operator1/1 -> READ FIFO/Enable
  Logical Operator4/1 -> READ IMU/Enable

== system TEST_LIDAR/HARDWARE/SENSORS/RCRX iBUS ==
  BUS UPDATE : MATLAB Function  Priority=20  TreatAsAtomicUnit=on
  Data Store Read19 : DataStoreRead  DataStoreName=CONTROL  SampleTime=SAMPLING_TIME  IndexOptions=Index vector (dialog)  Indices=1  OutputSizes=1
  Data Store Write1 : DataStoreWrite  DataStoreName=CONTROL  IndexOptions=Index vector (dialog)  Indices=1  OutputSizes=1
  Display3 : Display
  MATLAB Function : MATLAB Function  TreatAsAtomicUnit=on
  Serial Read1 : raspberrypiCommlib/Serial Read  board=Pi 3 Model B  SCIModule_=/dev/ttyS0  Baudrate_=115200  Parity=None  StopBits_=1  HardwareFlowControl=None  ByteOrder=LittleEndian  DataLength=70  DataType=uint8  OutputStatus=on  SampleTime=SAMPLING_TIME  blockPlatform=RaspberryPi
  Terminator : Terminator
  wires:
  MATLAB Function/1(CH_RAW) -> BUS UPDATE/2(CH_RAW)
  BUS UPDATE/1(CONTROL) -> Data Store Write1/1
  Data Store Read19/1 -> BUS UPDATE/1(CONTROL_IN)
  Serial Read1/1 -> MATLAB Function/1(iBUS_DATA), Display3/1
  Serial Read1/2 -> Terminator/1

== system TEST_LIDAR/HARDWARE/SENSORS/WALL RANGE SENSOR ==
  ANGLE AND DISTANCE COMPUTATION : Subsystem  TreatAsAtomicUnit=on
      settings: MinAlgLoopOccurrences=on
  Data Store Memory : DataStoreMemory  DataStoreName=REAR_DISTANCE  ReadBeforeWriteMsg=warning  WriteAfterWriteMsg=warning  WriteAfterReadMsg=warning  ShowAdditionalParam=off  OutDataTypeStr=double
  Data Store Memory1 : DataStoreMemory  DataStoreName=FRONT_DISTANCE  ReadBeforeWriteMsg=warning  WriteAfterWriteMsg=warning  WriteAfterReadMsg=warning  ShowAdditionalParam=off  OutDataTypeStr=double
  VL6180X_I2C_FRONT : Subsystem  TreatAsAtomicUnit=on
      settings: MinAlgLoopOccurrences=on  RTWSystemCode=Nonreusable function  FunctionWithSeparateData=on
  VL6180X_I2C_REAR : Subsystem  TreatAsAtomicUnit=on
      settings: MinAlgLoopOccurrences=on  RTWSystemCode=Nonreusable function  FunctionWithSeparateData=on

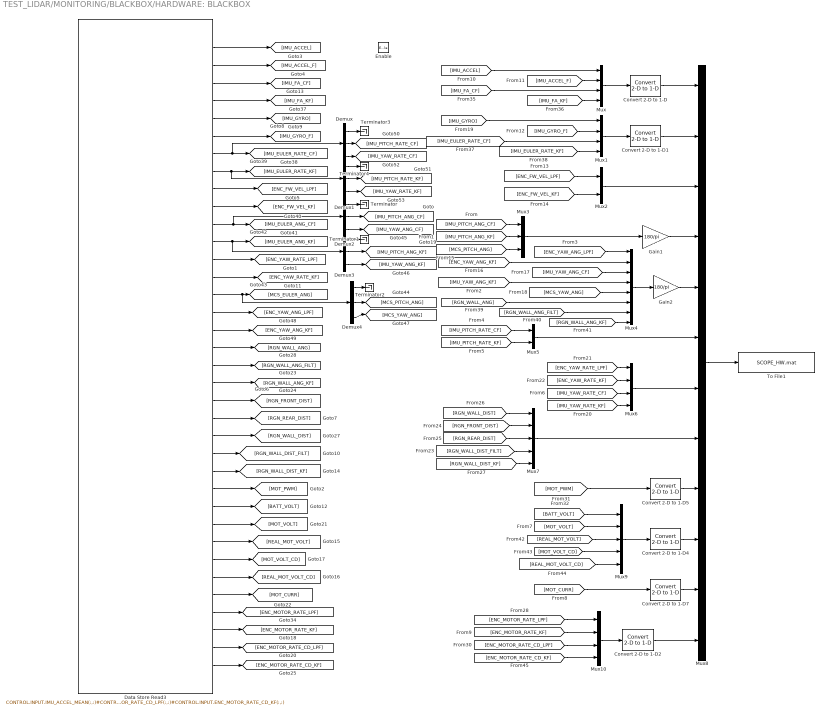
== system TEST_LIDAR/MONITORING/BLACKBOX/HARDWARE: BLACKBOX ==
  Enable : EnablePort
  Convert 2-D to 1-D{,1..2,4..5,7} (6 alike) : dspsigattribs/Convert 2-D to 1-D
  Data Store Read3 : DataStoreRead  DataStoreName=CONTROL  SampleTime=SAMPLING_TIME  DataStoreElements=CONTROL.INPUT.IMU_ACCEL_MEAN(:,:)#CONTROL.INPUT.IMU_ACCEL_MEAN_FILT(:,:)#CONTROL.INPUT.IMU_FORWARD_ACCEL_CF#CONTROL.INPUT.IMU_FORWARD_ACCEL_KF#CONTROL.INPUT.IMU_GYRO_MEAN(:,:)#CONTROL.INPUT.IMU_GYRO_MEAN_FILT(:,:)#CONTROL.INPUT.IMU_EULER_RATE_CF(:,:)#CONTROL.INPUT.IMU_EULER_RATE_KF(:,:)#CONTROL.INPUT.ENC_FORWARD_VEL_LPF#CONTROL.INPUT.ENC_FORWARD_VEL_KF#CONTROL.INPUT.IMU_EULER_ANG_CF(:,:)#CONTROL.INPUT.IMU_EULER_ANG_KF(:,:)#CONTROL.INPUT.ENC_YAW_RATE_LPF#CONTROL.INPUT.ENC_YAW_RATE_KF#CONTROL.INPUT.MCS_EULER_ANG(:,:)#CONTROL.INPUT.ENC_YAW_ANG_LPF#CONTROL.INPUT.ENC_YAW_ANG_KF#CONTROL.INPUT.RANGE_WALL_ANG#CONTROL.INPUT.WALL_ANG_FILT#CONTROL.INPUT.WALL_ANG_KF#CONTROL.INPUT.RANGE_FRONT_DIST#CONTROL.INPUT.RANGE_REAR_DIST#CONTROL.INPUT.RANGE_WALL_DIST#CONTROL.INPUT.WALL_DIST_FILT#CONTROL.INPUT.WALL_DIST_KF#CONTROL.OUTPUT.MOTOR_PWM(:,:)#CONTROL.INPUT.BATTERY_VOLT#CONTROL.OUTPUT.MOTOR_VOLT(:,:)#CONTROL.OUTPUT.REAL_MOTOR_VOLT(:,:)#CONTROL.OUTPUT.MOTOR_VOLT_CD(:,:)#CONTROL.OUTPUT.REAL_MOTOR_VOLT_CD(:,:)#CONTROL.INPUT.MOTOR_CURRENT(:,:)#CONTROL.INPUT.ENC_MOTOR_RATE_LPF(:,:)#CONTROL.INPUT.ENC_MOTOR_RATE_KF(:,:)#CONTROL.INPUT.ENC_MOTOR_RATE_CD_LPF(:,:)#CONTROL.INPUT.ENC_MOTOR_RATE_CD_KF(:,:)  IndexOptions=Index vector (dialog)  Indices=1  OutputSizes=1
  Demux{,1..4} (5 alike) : Demux  Outputs=3
  Gain1 : Gain  Gain=180/pi
  Gain2 : Gain  Gain=180/pi
  Mux{,1,6,10} (4 alike) : Mux
  Mux2 : Mux  Inputs=2
  Mux3 : Mux  Inputs=3
  Mux4 : Mux  Inputs=8
  Mux5 : Mux  Inputs=2
  Mux7 : Mux  Inputs=5
  Mux8 : Mux  Inputs=12
  Mux9 : Mux  Inputs=5
  Terminator{,1..4} (5 alike) : Terminator
  To File1 : ToFile  Filename=SCOPE_HW.mat  MatrixName=SCOPE_HW  SampleTime=SAMPLING_TIME
  wires:
  [MOT_CURR] -> Convert 2-D to 1-D7/1
  Convert 2-D to 1-D/1 -> Mux8/1
  Convert 2-D to 1-D1/1 -> Mux8/2
  Mux2/1 -> Mux8/3
  [IMU_ACCEL] -> Mux/1
  Mux/1 -> Convert 2-D to 1-D/1
  [IMU_ACCEL_F] -> Mux/2
  [ENC_FW_VEL_LPF] -> Mux2/1
  [ENC_FW_VEL_KF] -> Mux2/2
  [IMU_PITCH_ANG_CF] -> Mux3/1
  [IMU_PITCH_ANG_KF] -> Mux3/2
  Mux3/1 -> Gain1/1
  Gain1/1 -> Mux8/4
  Mux4/1 -> Gain2/1
  Gain2/1 -> Mux8/5
  Mux5/1 -> Mux8/6
  [IMU_PITCH_RATE_CF] -> Mux5/1
  [IMU_PITCH_RATE_KF] -> Mux5/2
  Mux6/1 -> Mux8/7
  Mux7/1 -> Mux8/8
  [RGN_WALL_DIST] -> Mux7/1
  [RGN_FRONT_DIST] -> Mux7/2
  [RGN_REAR_DIST] -> Mux7/3
  Mux9/1 -> Convert 2-D to 1-D4/1
  [MOT_VOLT] -> Mux9/2
  [BATT_VOLT] -> Mux9/1
  [MOT_PWM] -> Convert 2-D to 1-D5/1
  Convert 2-D to 1-D5/1 -> Mux8/9
  Convert 2-D to 1-D4/1 -> Mux8/10
  Convert 2-D to 1-D7/1 -> Mux8/11
  Data Store Read3/1 -> [IMU_ACCEL]
  Data Store Read3/2 -> [IMU_ACCEL_F]
  [ENC_MOTOR_RATE_KF] -> Mux10/2
  Mux10/1 -> Convert 2-D to 1-D2/1
  [ENC_MOTOR_RATE_LPF] -> Mux10/1
  Data Store Read3/32 -> [MOT_CURR]
  Data Store Read3/33 -> [ENC_MOTOR_RATE_LPF]
  Data Store Read3/34 -> [ENC_MOTOR_RATE_KF]
  Data Store Read3/5 -> [IMU_GYRO]
  Data Store Read3/6 -> [IMU_GYRO_F]
  Data Store Read3/3 -> [IMU_FA_CF]
  Data Store Read3/4 -> [IMU_FA_KF]
  [IMU_FA_CF] -> Mux/3
  [IMU_FA_KF] -> Mux/4
  Data Store Read3/7 -> Demux/1, [IMU_EULER_RATE_CF]
  Data Store Read3/8 -> Demux1/1, [IMU_EULER_RATE_KF]
  Mux1/1 -> Convert 2-D to 1-D1/1
  [IMU_GYRO] -> Mux1/1
  [IMU_GYRO_F] -> Mux1/2
  [IMU_EULER_RATE_CF] -> Mux1/3
  [IMU_EULER_RATE_KF] -> Mux1/4
  Data Store Read3/9 -> [ENC_FW_VEL_LPF]
  Data Store Read3/10 -> [ENC_FW_VEL_KF]
  Data Store Read3/11 -> Demux2/1, [IMU_EULER_ANG_CF]
  Data Store Read3/12 -> Demux3/1, [IMU_EULER_ANG_KF]
  Demux2/2 -> [IMU_PITCH_ANG_CF]
  Demux3/2 -> [IMU_PITCH_ANG_KF]
  Demux4/2 -> [MCS_PITCH_ANG]
  [MCS_PITCH_ANG] -> Mux3/3
  Demux2/3 -> [IMU_YAW_ANG_CF]
  Demux3/3 -> [IMU_YAW_ANG_KF]
  Demux2/1 -> Terminator/1
  Demux3/1 -> Terminator1/1
  Demux4/3 -> [MCS_YAW_ANG]
  Demux4/1 -> Terminator2/1
  [ENC_YAW_ANG_LPF] -> Mux4/1
  [ENC_YAW_ANG_KF] -> Mux4/2
  [IMU_YAW_ANG_CF] -> Mux4/3
  [IMU_YAW_ANG_KF] -> Mux4/4
  [MCS_YAW_ANG] -> Mux4/5
  [RGN_WALL_ANG] -> Mux4/6
  [RGN_WALL_ANG_FILT] -> Mux4/7
  [RGN_WALL_ANG_KF] -> Mux4/8
  Demux/2 -> [IMU_PITCH_RATE_CF]
  Demux1/2 -> [IMU_PITCH_RATE_KF]
  Demux/1 -> Terminator3/1
  Demux1/1 -> Terminator4/1
  Demux/3 -> [IMU_YAW_RATE_CF]
  Demux1/3 -> [IMU_YAW_RATE_KF]
  Data Store Read3/14 -> [ENC_YAW_RATE_KF]
  Data Store Read3/15 -> Demux4/1, [MCS_EULER_ANG]
  Data Store Read3/16 -> [ENC_YAW_ANG_LPF]
  Data Store Read3/17 -> [ENC_YAW_ANG_KF]
  Data Store Read3/18 -> [RGN_WALL_ANG]
  Data Store Read3/19 -> [RGN_WALL_ANG_FILT]
  Data Store Read3/20 -> [RGN_WALL_ANG_KF]
  Data Store Read3/13 -> [ENC_YAW_RATE_LPF]
  Data Store Read3/21 -> [RGN_FRONT_DIST]
  Data Store Read3/22 -> [RGN_REAR_DIST]
  Data Store Read3/23 -> [RGN_WALL_DIST]
  Data Store Read3/24 -> [RGN_WALL_DIST_FILT]
  Data Store Read3/25 -> [RGN_WALL_DIST_KF]
  [RGN_WALL_DIST_FILT] -> Mux7/4
  [RGN_WALL_DIST_KF] -> Mux7/5
  Data Store Read3/26 -> [MOT_PWM]
  Data Store Read3/27 -> [BATT_VOLT]
  Data Store Read3/28 -> [MOT_VOLT]
  Data Store Read3/29 -> [REAL_MOT_VOLT]
  Data Store Read3/31 -> [REAL_MOT_VOLT_CD]
  Data Store Read3/30 -> [MOT_VOLT_CD]
  [REAL_MOT_VOLT_CD] -> Mux9/5
  [REAL_MOT_VOLT] -> Mux9/3
  [MOT_VOLT_CD] -> Mux9/4
  Data Store Read3/35 -> [ENC_MOTOR_RATE_CD_LPF]
  Data Store Read3/36 -> [ENC_MOTOR_RATE_CD_KF]
  [ENC_MOTOR_RATE_CD_LPF] -> Mux10/3
  [ENC_MOTOR_RATE_CD_KF] -> Mux10/4
  Convert 2-D to 1-D2/1 -> Mux8/12
  [IMU_YAW_RATE_CF] -> Mux6/3
  [IMU_YAW_RATE_KF] -> Mux6/4
  [ENC_YAW_RATE_LPF] -> Mux6/1
  [ENC_YAW_RATE_KF] -> Mux6/2
  Mux8/1 -> To File1/1

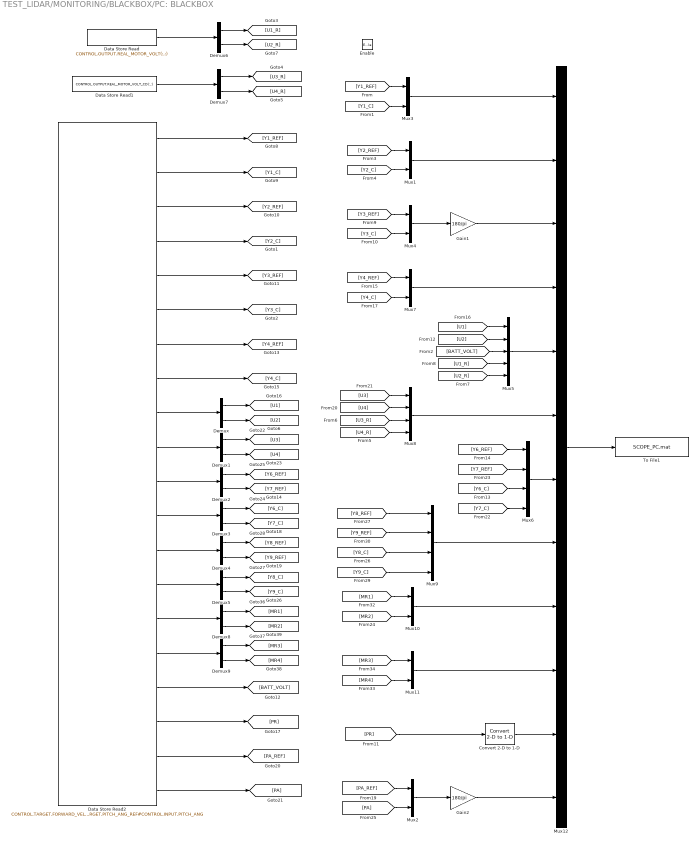
== system TEST_LIDAR/MONITORING/BLACKBOX/PC: BLACKBOX ==
  Enable : EnablePort
  Convert 2-D to 1-D : dspsigattribs/Convert 2-D to 1-D
  Data Store Read : DataStoreRead  DataStoreName=CONTROL  DataStoreElements=CONTROL.OUTPUT.REAL_MOTOR_VOLT(:,:)  IndexOptions=Index vector (dialog)  Indices=1  OutputSizes=1
  Data Store Read1 : DataStoreRead  DataStoreName=CONTROL  DataStoreElements=CONTROL.OUTPUT.REAL_MOTOR_VOLT_CD(:,:)  IndexOptions=Index vector (dialog)  Indices=1  OutputSizes=1
  Data Store Read2 : DataStoreRead  DataStoreName=CONTROL  SampleTime=SAMPLING_TIME  DataStoreElements=CONTROL.TARGET.FORWARD_VEL_REF#CONTROL.INPUT.FORWARD_VEL#CONTROL.TARGET.YAW_RATE_REF#CONTROL.INPUT.YAW_RATE#CONTROL.TARGET.YAW_ANG_REF#CONTROL.INPUT.YAW_ANG#CONTROL.TARGET.WALL_DIST_REF#CONTROL.INPUT.WALL_DIST#CONTROL.OUTPUT.MOTOR_VOLT(:,:)#CONTROL.OUTPUT.MOTOR_VOLT_CD(:,:)#CONTROL.TARGET.POS_XY_REF(:,:)#CONTROL.INPUT.EARTH_POS(1:2,1)#CONTROL.TARGET.VEL_XY_REF(:,:)#CONTROL.INPUT.EARTH_VEL(1:2,1)#CONTROL.INPUT.MOTOR_RATE(:,:)#CONTROL.INPUT.MOTOR_RATE_CD(:,:)#CONTROL.INPUT.BATTERY_VOLT#CONTROL.INPUT.PITCH_RATE#CONTROL.TARGET.PITCH_ANG_REF#CONTROL.INPUT.PITCH_ANG  IndexOptions=Index vector (dialog)  Indices=1  OutputSizes=1
  Demux{,1..9} (10 alike) : Demux  Outputs=2
  Gain1 : Gain  Gain=180/pi
  Gain2 : Gain  Gain=180/pi
  Mux{1..4,7,10..11} (7 alike) : Mux  Inputs=2
  Mux12 : Mux  Inputs=12
  Mux5 : Mux  Inputs=5
  Mux6 : Mux
  Mux8 : Mux
  Mux9 : Mux
  To File1 : ToFile  Filename=SCOPE_PC.mat  MatrixName=SCOPE_PC  SampleTime=SAMPLING_TIME
  wires:
  Gain2/1 -> Mux12/12
  Data Store Read2/17 -> [BATT_VOLT]
  [PR] -> Convert 2-D to 1-D/1
  Data Store Read2/7 -> [Y4_REF]
  Data Store Read2/5 -> [Y3_REF]
  [Y4_C] -> Mux7/2
  Data Store Read2/1 -> [Y1_REF]
  Data Store Read2/14 -> Demux5/1
  Demux8/1 -> [MR1]
  Data Store Read2/4 -> [Y2_C]
  Data Store Read2/2 -> [Y1_C]
  [MR1] -> Mux10/1
  Demux7/2 -> [U4_R]
  [Y9_C] -> Mux9/4
  Demux5/2 -> [Y9_C]
  [PA] -> Mux2/2
  [U4] -> Mux8/2
  [MR3] -> Mux11/1
  Demux1/2 -> [U4]
  Data Store Read2/16 -> Demux9/1
  Demux4/2 -> [Y9_REF]
  Data Store Read2/8 -> [Y4_C]
  [Y1_C] -> Mux3/2
  [Y1_REF] -> Mux3/1
  [U2] -> Mux5/2
  Demux/2 -> [U2]
  Mux1/1 -> Mux12/2
  Demux7/1 -> [U3_R]
  [Y9_REF] -> Mux9/2
  Data Store Read2/18 -> [PR]
  Demux6/1 -> [U1_R]
  Mux9/1 -> Mux12/8
  [Y7_C] -> Mux6/4
  [Y2_C] -> Mux1/2
  Mux6/1 -> Mux12/7
  Mux12/1 -> To File1/1
  Demux2/2 -> [Y7_REF]
  Data Store Read2/12 -> Demux3/1
  Data Store Read2/9 -> Demux/1
  [Y3_C] -> Mux4/2
  [Y2_REF] -> Mux1/1
  Data Store Read2/15 -> Demux8/1
  Mux3/1 -> Mux12/1
  [MR4] -> Mux11/2
  Mux10/1 -> Mux12/9
  [Y6_C] -> Mux6/3
  Data Store Read2/10 -> Demux1/1
  Mux4/1 -> Gain1/1
  Demux1/1 -> [U3]
  [Y8_REF] -> Mux9/1
  Data Store Read/1 -> Demux6/1
  Demux4/1 -> [Y8_REF]
  Demux3/2 -> [Y7_C]
  Demux2/1 -> [Y6_REF]
  Demux3/1 -> [Y6_C]
  [Y3_REF] -> Mux4/1
  [PA_REF] -> Mux2/1
  [Y6_REF] -> Mux6/1
  Data Store Read2/11 -> Demux2/1
  [U3_R] -> Mux8/3
  Demux6/2 -> [U2_R]
  Mux5/1 -> Mux12/5
  Mux8/1 -> Mux12/6
  Demux8/2 -> [MR2]
  Gain1/1 -> Mux12/3
  [Y7_REF] -> Mux6/2
  Mux7/1 -> Mux12/4
  Data Store Read2/13 -> Demux4/1
  Data Store Read2/19 -> [PA_REF]
  Demux/1 -> [U1]
  [U4_R] -> Mux8/4
  [U1_R] -> Mux5/4
  Mux2/1 -> Gain2/1
  Convert 2-D to 1-D/1 -> Mux12/11
  Demux5/1 -> [Y8_C]
  [Y4_REF] -> Mux7/1
  Demux9/2 -> [MR4]
  Data Store Read2/6 -> [Y3_C]
  Mux11/1 -> Mux12/10
  [U2_R] -> Mux5/5
  Data Store Read1/1 -> Demux7/1
  Data Store Read2/3 -> [Y2_REF]
  [U1] -> Mux5/1
  Demux9/1 -> [MR3]
  [Y8_C] -> Mux9/3
  Data Store Read2/20 -> [PA]
  [U3] -> Mux8/1
  [BATT_VOLT] -> Mux5/3
  [MR2] -> Mux10/2
